simulink model "P4_Model_Final"  (R2023b)
settings: Solver=VariableStepAuto  StartTime=0.0  StopTime=3600  RelTol=1e-3
values from neighbouring files (symbols this model uses):
  C0 = 0.0041    [P4initUpdated.m]
  C1 = 0.000066    (= 6.6e-05)    [P4initUpdated.m]
  C2 = 0.5*Rho*A*Cd    (= 0.51156)    [P4initUpdated.m]
  Iw = 0.5*7*(r^2)    (= 0.4536)    [P4initUpdated.m]
  M = 1000    [P4initUpdated.m]
  r = 0.36    [P4initUpdated.m]
  rps2rpm = 60/(2*pi())    [P4initUpdated.m]
  Wp = [transpose(x), transpose(y)]    [genTrack.m]
undefined symbols (not defined in the file or in its folder): batData, carData, motorData
libraries: slpidlib x2
settings Model: Creator=jessi  LastModifiedBy=lmend

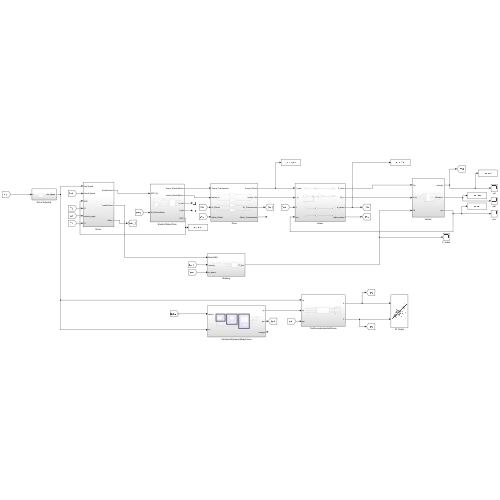
[thumbnail: Simulink's stored preview of the top-level diagram]
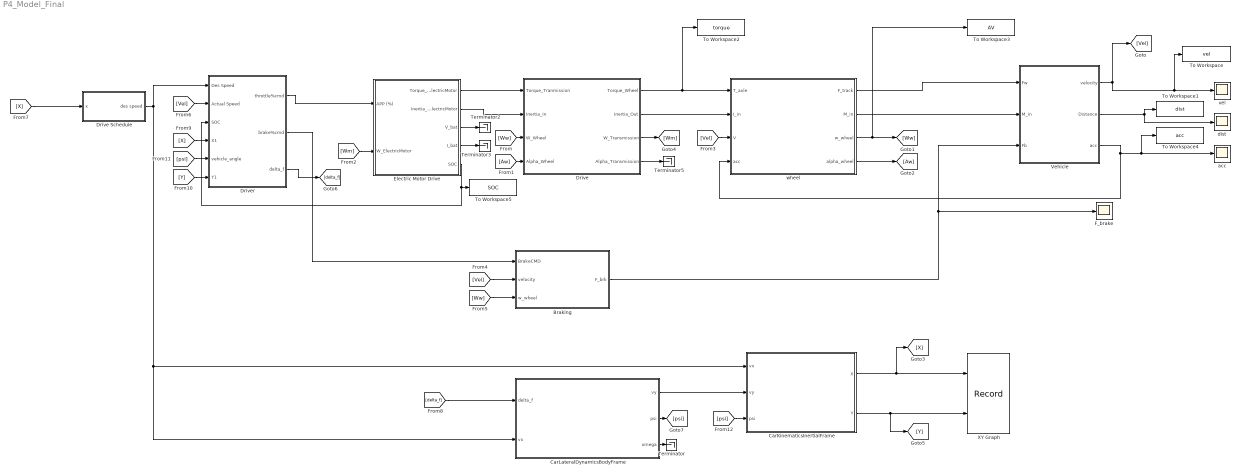
== system P4_Model_Final ==
  Braking : Subsystem
  CarKinematicsInertialFrame : Subsystem
  CarLateralDynamicsBodyFrame : Subsystem
  Drive : Subsystem
  Drive Schedule : Subsystem
  Driver : Subsystem
  Electric Motor Drive : Subsystem
  F_brake : Scope
  Terminator{,2..3,5} (4 alike) : Terminator
  To Workspace : ToWorkspace  VariableName=vel  SaveFormat=Timeseries  SampleTime=-1
  To Workspace1 : ToWorkspace  VariableName=dist  SaveFormat=Timeseries  SampleTime=-1
  To Workspace2 : ToWorkspace  VariableName=torque  SaveFormat=Timeseries  SampleTime=-1
  To Workspace3 : ToWorkspace  VariableName=AV  SaveFormat=Timeseries  SampleTime=-1
  To Workspace4 : ToWorkspace  VariableName=acc  SaveFormat=Timeseries  SampleTime=-1
  To Workspace5 : ToWorkspace  VariableName=SOC  SaveFormat=Timeseries  SampleTime=-1
  Vehicle : Subsystem
  XY Graph : Record  FileSettingsInternal="{\"entries\":[{\"content\":{\"excelSettings\":{\"content\":{},\"type\":\"Streamout.ExcelSettings\"}},\"type\":\"Streamout.FileSettingStorage\",\"uuid\":\"\"}],\"packageUris\":[\"http:\\/\\/schema.mathworks.com\\/mf0\\/streamout_blocks\\/R2020a\"],\"version\":\"1.0\"}"  Layout=[1 1]  SignalsInternal="{\"entries\":[{\"content\":{\"signals\":[{\"content\":{\"blockPath\":[],\"dimensions\":[1],\"domain\":\"\",\"lineColor\":\"#7e2f8e\",\"port\":1,\"sid\":[\"\"],\"signalID\":5613,\"signalName\":\"CarKinematicsInertialFrame:1\"},\"type\":\"RecordBlkView.Signal\",\"uuid\":\"\"},{\"content\":{\"blockPath\":[],\"dimensions\":[1],\"domain\":\"\",\"lineColor\":\"#77ac30\",\"port\":2,\"sid\":[\"\"],\"signalID\":5617,\"signalName\":\"CarKinematicsInertialFrame:2\"},\"type\":\"RecordBlkView.Signal\",\"uuid\":\"\"}]},\"type\":\"RecordBlkView.InputSignals\",\"uuid\":\"\"}],\"packageUris\":[\"http:\\/\\/schema.mathworks.com\\/mf0\\/streamout_blocks\\/R2020a\"],\"version\":\"1.0\"}"  VisualizationBindings="{\"xyplotplugin\":{\"info\":[{\"series\":[],\"subplotID\":1}]}}"  CompatibilityTag=XY  st=-1
  acc : Scope
  dist : Scope
  vel : Scope
  "wheel " : Subsystem
  wires:
  [Ww] -> Braking/3(w_wheel)
  [Vel] -> Braking/2("velocity ")
  "wheel "/3(w_wheel) -> To Workspace3/1, [Ww]
  "wheel "/1(F_track) -> Vehicle/1("Fw ")
  [Wm] -> Electric Motor Drive/2(W_ElectricMotor)
  "wheel "/2(M_in) -> Vehicle/2("M_in ")
  [Ww] -> Drive/3(W_Wheel)
  Drive/1(Torque_Wheel) -> To Workspace2/1, "wheel "/1(T_axle)
  Drive/2(Inertia_Out) -> "wheel "/2(I_in)
  Electric Motor Drive/4(I_bat) -> Terminator3/1
  [Vel] -> "wheel "/3(V)
  Electric Motor Drive/3(V_bat) -> Terminator2/1
  Vehicle/2("Distance ") -> dist/1, To Workspace1/1
  Braking/1("F_brk ") -> F_brake/1, Vehicle/3("Fb ")
  Drive/4(Alpha_Transmission) -> Terminator5/1
  Electric Motor Drive/2(Inertia_ElectricMotor) -> Drive/2(Inertia_In)
  Vehicle/3(acc) -> "wheel "/4(acc), To Workspace4/1, acc/1
  Vehicle/1("velocity ") -> To Workspace/1, vel/1, [Vel]
  Electric Motor Drive/1(Torque_ElectricMotor) -> Drive/1(Torque_Tranmission)
  "wheel "/4(alpha_wheel) -> [Aw]
  [Aw] -> Drive/4(Alpha_Wheel)
  Drive/3(W_Transmission) -> [Wm]
  Drive Schedule/1("des speed ") -> Driver/1("Des Speed "), CarKinematicsInertialFrame/1(vx), CarLateralDynamicsBodyFrame/2(vx)
  [delta_f] -> CarLateralDynamicsBodyFrame/1(delta_f)
  CarKinematicsInertialFrame/1(X) -> [X], XY Graph/1
  CarKinematicsInertialFrame/2(Y) -> [Y], XY Graph/2
  CarLateralDynamicsBodyFrame/1(vy) -> CarKinematicsInertialFrame/2(vy)
  [X] -> Drive Schedule/1(x)
  CarLateralDynamicsBodyFrame/3(omega) -> Terminator/1
  [Y] -> Driver/6(Y1)
  Driver/3(delta_f) -> [delta_f]
  Driver/2("brake%cmd ") -> Braking/1("BrakeCMD ")
  Driver/1(throttle%cmd) -> Electric Motor Drive/1(APP (%))
  CarLateralDynamicsBodyFrame/2(psi) -> [psi]
  [psi] -> CarKinematicsInertialFrame/3(psi)
  Electric Motor Drive/5(SOC) -> Driver/3(SOC), To Workspace5/1
  [X] -> Driver/4(X1)
  [Vel] -> Driver/2(Actual Speed)
  [psi] -> Driver/5(vehicle_angle)

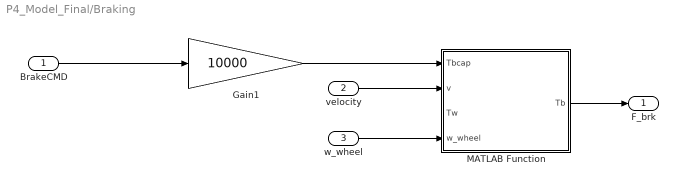
== system P4_Model_Final/Braking ==
  "BrakeCMD " : Inport
  "velocity " : Inport  Port=2
  w_wheel : Inport  Port=3
  Gain1 : Gain  Gain=10000
  MATLAB Function : MATLAB Function  TreatAsAtomicUnit=on
  "F_brk " : Outport  VectorParamsAs1DForOutWhenUnconnected=off
  wires:
  "BrakeCMD "/1 -> Gain1/1
  Gain1/1 -> MATLAB Function/1(Tbcap)
  MATLAB Function/1(Tb) -> "F_brk "/1
  "velocity "/1 -> MATLAB Function/2(v)
  w_wheel/1 -> MATLAB Function/4(w_wheel)

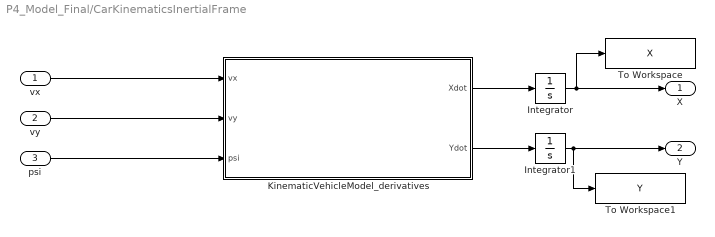
== system P4_Model_Final/CarKinematicsInertialFrame ==
  vx : Inport
  vy : Inport  Port=2
  psi : Inport  Port=3
  Integrator : Integrator  InitialCondition=carData.init.X0
  Integrator1 : Integrator  InitialCondition=carData.init.Y0
  KinematicVehicleModel_derivatives : MATLAB Function  TreatAsAtomicUnit=on  mask{obj=carData}
      mask prompts: obj "obj structure"
  To Workspace : ToWorkspace  VariableName=X  SaveFormat=Timeseries  SampleTime=-1
  To Workspace1 : ToWorkspace  VariableName=Y  SaveFormat=Timeseries  SampleTime=-1
  X : Outport
  Y : Outport  Port=2
  wires:
  KinematicVehicleModel_derivatives/1(Xdot) -> Integrator/1
  KinematicVehicleModel_derivatives/2(Ydot) -> Integrator1/1
  Integrator/1 -> To Workspace/1, X/1
  Integrator1/1 -> To Workspace1/1, Y/1
  vx/1 -> KinematicVehicleModel_derivatives/1(vx)
  vy/1 -> KinematicVehicleModel_derivatives/2(vy)
  psi/1 -> KinematicVehicleModel_derivatives/3(psi)

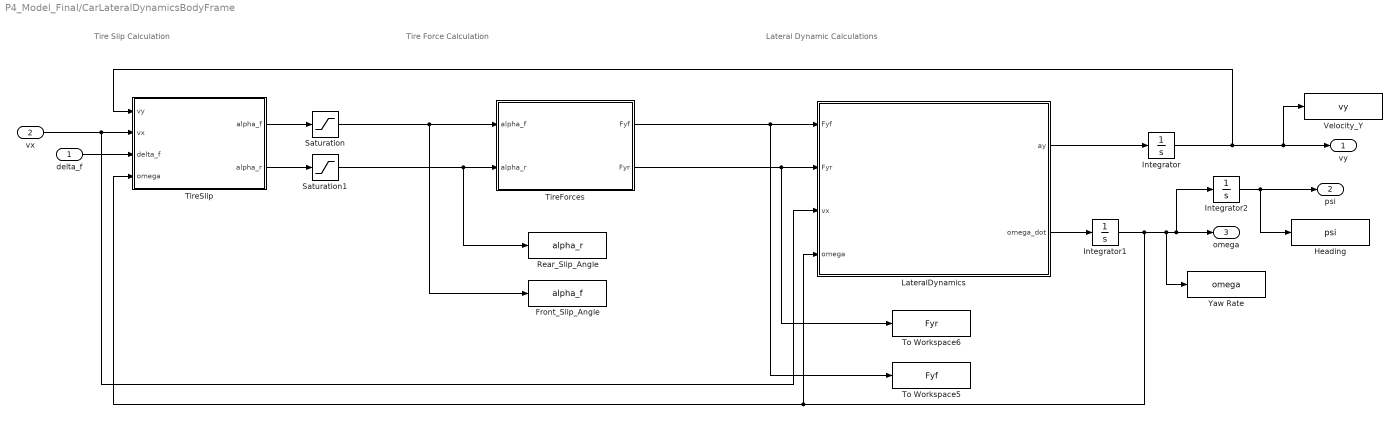
== system P4_Model_Final/CarLateralDynamicsBodyFrame ==
  note: Tire Slip Calculation
  note: Tire Force Calculation
  note: Lateral Dynamic Calculations
  delta_f : Inport
  vx : Inport  Port=2
  Front_Slip_Angle : ToWorkspace  VariableName=alpha_f  SaveFormat=Timeseries  SampleTime=-1
  Heading : ToWorkspace  VariableName=psi  SaveFormat=Timeseries  SampleTime=-1
  Integrator : Integrator  InitialCondition=carData.init.vy0
  Integrator1 : Integrator  InitialCondition=carData.init.omega0
  Integrator2 : Integrator  InitialCondition=carData.init.psi0
  LateralDynamics : MATLAB Function  TreatAsAtomicUnit=on  mask{obj=carData}
      mask prompts: obj "obj structure"
  Rear_Slip_Angle : ToWorkspace  VariableName=alpha_r  SaveFormat=Timeseries  SampleTime=-1
  Saturation : Saturate  UpperLimit=carData.maxAlpha  LowerLimit=-carData.maxAlpha
  Saturation1 : Saturate  UpperLimit=carData.maxAlpha  LowerLimit=-carData.maxAlpha
  TireForces : MATLAB Function  TreatAsAtomicUnit=on  mask{obj=carData}
      mask prompts: obj "obj structure"
  TireSlip : MATLAB Function  TreatAsAtomicUnit=on  mask{obj=carData}
      mask prompts: obj "obj structure"
  To Workspace5 : ToWorkspace  VariableName=Fyf  SaveFormat=Timeseries  SampleTime=-1
  To Workspace6 : ToWorkspace  VariableName=Fyr  SaveFormat=Timeseries  SampleTime=-1
  Velocity_Y : ToWorkspace  VariableName=vy  SaveFormat=Timeseries  SampleTime=-1
  Yaw Rate : ToWorkspace  VariableName=omega  SaveFormat=Timeseries  SampleTime=-1
  vy : Outport
  psi : Outport  Port=2
  omega : Outport  Port=3
  wires:
  LateralDynamics/1(ay) -> Integrator/1
  Integrator/1 -> vy/1, Velocity_Y/1, TireSlip/1(vy)
  LateralDynamics/2(omega_dot) -> Integrator1/1
  Integrator1/1 -> Integrator2/1, omega/1, Yaw Rate/1, LateralDynamics/4(omega), TireSlip/4(omega)
  TireSlip/1(alpha_f) -> Saturation/1
  TireSlip/2(alpha_r) -> Saturation1/1
  TireForces/1(Fyf) -> LateralDynamics/1(Fyf), To Workspace5/1
  TireForces/2(Fyr) -> LateralDynamics/2(Fyr), To Workspace6/1
  Saturation/1 -> TireForces/1(alpha_f), Front_Slip_Angle/1
  Saturation1/1 -> TireForces/2(alpha_r), Rear_Slip_Angle/1
  vx/1 -> TireSlip/2(vx), LateralDynamics/3(vx)
  delta_f/1 -> TireSlip/3(delta_f)
  Integrator2/1 -> Heading/1, psi/1

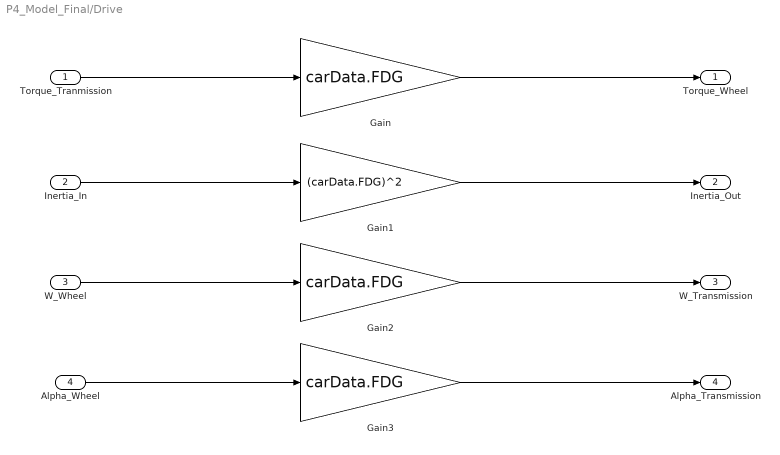
== system P4_Model_Final/Drive ==
  Torque_Tranmission : Inport
  Inertia_In : Inport  Port=2
  W_Wheel : Inport  Port=3
  Alpha_Wheel : Inport  Port=4
  Gain : Gain  Gain=carData.FDG
  Gain1 : Gain  Gain=(carData.FDG)^2
  Gain2 : Gain  Gain=carData.FDG
  Gain3 : Gain  Gain=carData.FDG
  Torque_Wheel : Outport
  Inertia_Out : Outport  Port=2
  W_Transmission : Outport  Port=3
  Alpha_Transmission : Outport  Port=4
  wires:
  Torque_Tranmission/1 -> Gain/1
  Inertia_In/1 -> Gain1/1
  W_Wheel/1 -> Gain2/1
  Alpha_Wheel/1 -> Gain3/1
  Gain/1 -> Torque_Wheel/1
  Gain1/1 -> Inertia_Out/1
  Gain2/1 -> W_Transmission/1
  Gain3/1 -> Alpha_Transmission/1

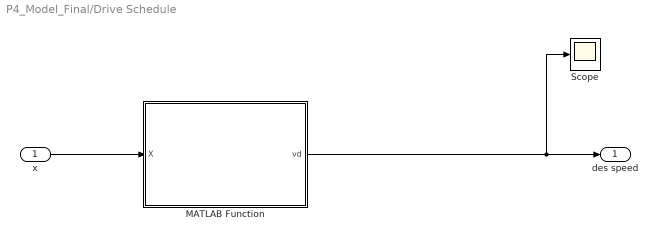
== system P4_Model_Final/Drive Schedule ==
  x : Inport
  MATLAB Function : MATLAB Function  TreatAsAtomicUnit=on
  Scope : Scope
  "des speed " : Outport  VectorParamsAs1DForOutWhenUnconnected=off
  wires:
  x/1 -> MATLAB Function/1(X)
  MATLAB Function/1(vd) -> "des speed "/1, Scope/1

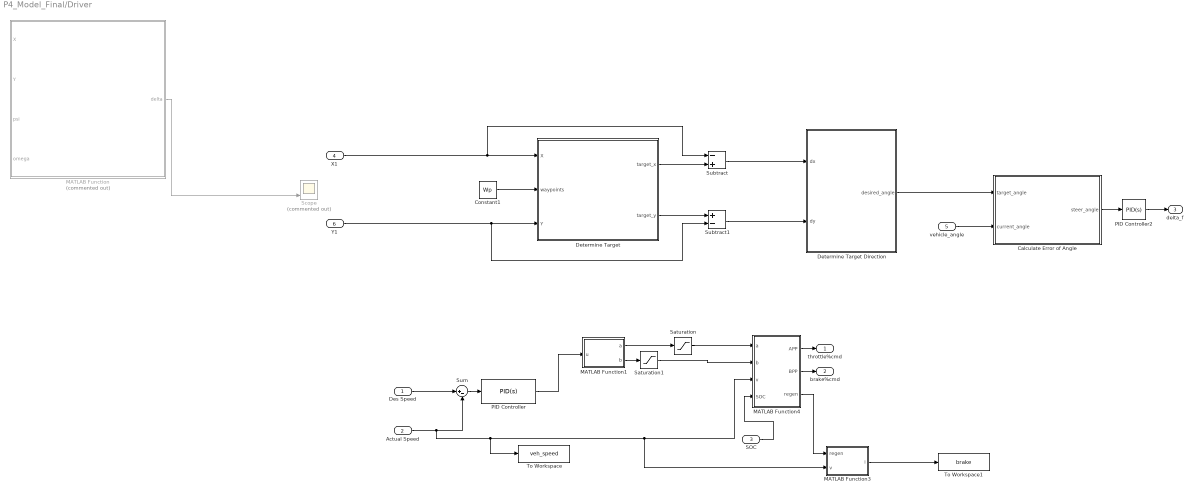
== system P4_Model_Final/Driver ==
  "Des Speed " : Inport
  Actual Speed : Inport  Port=2
  SOC : Inport  Port=3
  X1 : Inport  Port=4
  vehicle_angle : Inport  Port=5
  Y1 : Inport  Port=6
  Calculate Error of Angle : MATLAB Function  TreatAsAtomicUnit=on
  Constant1 : Constant  Value=Wp
  Determine Target : MATLAB Function  TreatAsAtomicUnit=on
  Determine Target Direction : MATLAB Function  TreatAsAtomicUnit=on
  MATLAB Function : MATLAB Function  Commented=on  TreatAsAtomicUnit=on
  MATLAB Function1 : MATLAB Function  TreatAsAtomicUnit=on
  MATLAB Function3 : MATLAB Function  TreatAsAtomicUnit=on
  MATLAB Function4 : MATLAB Function  TreatAsAtomicUnit=on
  PID Controller : slpidlib/PID Controller  Controller=PID  Form=Parallel  TimeDomain=Continuous-time  UseExternalTs=off  SampleTime=-1  IntegratorMethod=Forward Euler  FilterMethod=Forward Euler  ControllerParametersSource=internal  P=0.55  I=0  UseKiTs=off  D=0  N=100  UseFilter=on  TunerSelectOption=Transfer Function Based (PID Tuner App)  InitialConditionSource=internal  InitialConditionForIntegrator=0  InitialConditionForFilter=0  DifferentiatorICPrevScaledInput=0  ExternalReset=none  TrackingMode=off  Kt=1  LimitOutput=on  SatLimitsSource=internal  UpperSaturationLimit=1  LowerSaturationLimit=-1  LinearizeAsGain=off  AntiWindupMode=none  Kb=1  LimitIntegrator=off  UpperIntegratorSaturationLimit=inf  LowerIntegratorSaturationLimit=-inf  POutMin=[]  POutMax=[]  IOutMin=[]  IOutMax=[]  DOutMin=[]  DOutMax=[]  NOutMin=[]  NOutMax=[]  SumOutMin=[]  SumOutMax=[]  SaturationOutMin=[]  SaturationOutMax=[]  PParamMin=[]  PParamMax=[]  IParamMin=[]  IParamMax=[]  DParamMin=[]  DParamMax=[]  NParamMin=[]  NParamMax=[]  KbParamMin=[]  KbParamMax=[]  KtParamMin=[]  KtParamMax=[]  KbOutMin=[]  KbOutMax=[]  KtOutMin=[]  KtOutMax=[]  IntegratorOutMin=[]  IntegratorOutMax=[]  FilterOutMin=[]  FilterOutMax=[]  SumI1OutMin=[]  SumI1OutMax=[]  SumI2OutMin=[]  SumI2OutMax=[]  SumI3OutMin=[]  SumI3OutMax=[]  SumI4OutMin=[]  SumI4OutMax=[]  SumDOutMin=[]  SumDOutMax=[]  DifferentiatorOutMin=[]  DifferentiatorOutMax=[]  FilterDiffOutCoefMin=[]  FilterDiffOutCoefMax=[]  ReciprocalOutMin=[]  ReciprocalOutMax=[]  SumDenOutMin=[]  SumDenOutMax=[]  SumNumOutMin=[]  SumNumOutMax=[]  DivideOutMin=[]  DivideOutMax=[]  UdiffTsProdOutMin=[]  UdiffTsProdOutMax=[]  NTsProdOutMin=[]  NTsProdOutMax=[]  UintegralTsProdOutMin=[]  UintegralTsProdOutMax=[]  UngainTsProdOutMin=[]  UngainTsProdOutMax=[]  ClampingZeroOutDataTypeStr=Inherit: Inherit via back propagation  ClampingZeroOutMin=[]  ClampingZeroOutMax=[]  FilterDenConstantOutDataTypeStr=Inherit: Inherit via back propagation  FilterDenConstantOutMin=[]  FilterDenConstantOutMax=[]  PCopyOutDataTypeStr=Inherit: Inherit via back propagation  PCopyOutMin=[]  PCopyOutMax=[]  NCopyOutDataTypeStr=Inherit: Inherit via back propagation  NCopyOutMin=[]  NCopyOutMax=[]  IntegratorContinuousStateAttributes=''  IntegratorStateMustResolveToSignalObject=off  IntegratorRTWStateStorageClass=Auto  FilterContinuousStateAttributes=''  FilterStateMustResolveToSignalObject=off  FilterRTWStateStorageClass=Auto  ParallelPVariant=InternalParameters  IdealPVariant=Disabled  IVariant=InternalParameters  DVariant=InternalParameters  IntegratorVariant=Continuous  SatVariant=Enabled  AWVariant=Passthrough  PCopyVariant=Disabled  TRVariant=Disabled  FdbkBlocksVariant=Forward  IdealPFdbkVariant=Disabled  SatFdbkVariant=Disabled  DerivativeFilterVariant=ContFilter  NVariant=InternalParameters  NCopyVariant=Disabled  FilterICVariant=InternalICsFilter  IntegratorICVariant=InternalICs  ExternalResetVariant=Disabled  TRSumVariant=Passthrough  SumFdbkVariant=Disabled  SumVariant=Sum_PID  TsampFilterVariant=InternalTs  TsampNgainVariant=Passthrough  TsampIntegralVariant=Disabled_SignalSpec  ExternalSaturationOutDataTypeStr=Inherit: Same as second input
  PID Controller2 : slpidlib/PID Controller  Controller=PID  Form=Parallel  TimeDomain=Continuous-time  UseExternalTs=off  SampleTime=-1  IntegratorMethod=Forward Euler  FilterMethod=Forward Euler  ControllerParametersSource=internal  P=1  I=0.1  UseKiTs=off  D=0  N=100  UseFilter=on  TunerSelectOption=Transfer Function Based (PID Tuner App)  InitialConditionSource=internal  InitialConditionForIntegrator=0  InitialConditionForFilter=0  DifferentiatorICPrevScaledInput=0  ExternalReset=none  TrackingMode=off  Kt=1  LimitOutput=off  SatLimitsSource=internal  UpperSaturationLimit=inf  LowerSaturationLimit=-inf  LinearizeAsGain=on  AntiWindupMode=none  Kb=1  LimitIntegrator=off  UpperIntegratorSaturationLimit=inf  LowerIntegratorSaturationLimit=-inf  POutMin=[]  POutMax=[]  IOutMin=[]  IOutMax=[]  DOutMin=[]  DOutMax=[]  NOutMin=[]  NOutMax=[]  SumOutMin=[]  SumOutMax=[]  SaturationOutMin=[]  SaturationOutMax=[]  PParamMin=[]  PParamMax=[]  IParamMin=[]  IParamMax=[]  DParamMin=[]  DParamMax=[]  NParamMin=[]  NParamMax=[]  KbParamMin=[]  KbParamMax=[]  KtParamMin=[]  KtParamMax=[]  KbOutMin=[]  KbOutMax=[]  KtOutMin=[]  KtOutMax=[]  IntegratorOutMin=[]  IntegratorOutMax=[]  FilterOutMin=[]  FilterOutMax=[]  SumI1OutMin=[]  SumI1OutMax=[]  SumI2OutMin=[]  SumI2OutMax=[]  SumI3OutMin=[]  SumI3OutMax=[]  SumI4OutMin=[]  SumI4OutMax=[]  SumDOutMin=[]  SumDOutMax=[]  DifferentiatorOutMin=[]  DifferentiatorOutMax=[]  FilterDiffOutCoefMin=[]  FilterDiffOutCoefMax=[]  ReciprocalOutMin=[]  ReciprocalOutMax=[]  SumDenOutMin=[]  SumDenOutMax=[]  SumNumOutMin=[]  SumNumOutMax=[]  DivideOutMin=[]  DivideOutMax=[]  UdiffTsProdOutMin=[]  UdiffTsProdOutMax=[]  NTsProdOutMin=[]  NTsProdOutMax=[]  UintegralTsProdOutMin=[]  UintegralTsProdOutMax=[]  UngainTsProdOutMin=[]  UngainTsProdOutMax=[]  ClampingZeroOutDataTypeStr=Inherit: Inherit via back propagation  ClampingZeroOutMin=[]  ClampingZeroOutMax=[]  FilterDenConstantOutDataTypeStr=Inherit: Inherit via back propagation  FilterDenConstantOutMin=[]  FilterDenConstantOutMax=[]  PCopyOutDataTypeStr=Inherit: Inherit via back propagation  PCopyOutMin=[]  PCopyOutMax=[]  NCopyOutDataTypeStr=Inherit: Inherit via back propagation  NCopyOutMin=[]  NCopyOutMax=[]  IntegratorContinuousStateAttributes=''  IntegratorStateMustResolveToSignalObject=off  IntegratorRTWStateStorageClass=Auto  FilterContinuousStateAttributes=''  FilterStateMustResolveToSignalObject=off  FilterRTWStateStorageClass=Auto  ParallelPVariant=InternalParameters  IdealPVariant=Disabled  IVariant=InternalParameters  DVariant=InternalParameters  IntegratorVariant=Continuous  SatVariant=Disabled  AWVariant=Passthrough  PCopyVariant=Disabled  TRVariant=Disabled  FdbkBlocksVariant=Forward  IdealPFdbkVariant=Disabled  SatFdbkVariant=Disabled  DerivativeFilterVariant=ContFilter  NVariant=InternalParameters  NCopyVariant=Disabled  FilterICVariant=InternalICsFilter  IntegratorICVariant=InternalICs  ExternalResetVariant=Disabled  TRSumVariant=Passthrough  SumFdbkVariant=Disabled  SumVariant=Sum_PID  TsampFilterVariant=InternalTs  TsampNgainVariant=Passthrough  TsampIntegralVariant=Disabled_SignalSpec  ExternalSaturationOutDataTypeStr=Inherit: Same as second input
  Saturation : Saturate  UpperLimit=1  LowerLimit=0
  Saturation1 : Saturate  UpperLimit=0  LowerLimit=-1
  Scope : Scope  Commented=on  NumInputPorts=3
  Subtract : Sum  Inputs=-+
  Subtract1 : Sum  Inputs=+-
  Sum : Sum  Inputs=|+-
  To Workspace : ToWorkspace  VariableName=veh_speed  SaveFormat=Timeseries  SampleTime=-1
  To Workspace1 : ToWorkspace  VariableName=brake  SaveFormat=Timeseries  SampleTime=-1
  throttle%cmd : Outport
  "brake%cmd " : Outport  Port=2
  delta_f : Outport  Port=3
  wires:
  MATLAB Function/1(delta) -> Scope/3
  PID Controller/1 -> MATLAB Function1/1(u)
  MATLAB Function1/2(b) -> Saturation1/1
  Actual Speed/1 -> To Workspace/1, MATLAB Function3/2(v), MATLAB Function4/3(v), Sum/2
  Sum/1 -> PID Controller/1
  MATLAB Function1/1(a) -> Saturation/1
  "Des Speed "/1 -> Sum/1
  MATLAB Function3/1(i) -> To Workspace1/1
  MATLAB Function4/2(BPP) -> "brake%cmd "/1
  MATLAB Function4/1(APP) -> throttle%cmd/1
  MATLAB Function4/3(regen) -> MATLAB Function3/1(regen)
  Saturation/1 -> MATLAB Function4/1(a)
  Saturation1/1 -> MATLAB Function4/2(b)
  SOC/1 -> MATLAB Function4/4(SOC)
  Determine Target/1(target_x) -> Subtract/2
  Y1/1 -> Subtract1/2, Determine Target/3(Y)
  Subtract1/1 -> Determine Target Direction/2(dy)
  Determine Target Direction/1(desired_angle) -> Calculate Error of Angle/1(target_angle)
  Determine Target/2(target_y) -> Subtract1/1
  Constant1/1 -> Determine Target/2(waypoints)
  Subtract/1 -> Determine Target Direction/1(dx)
  PID Controller2/1 -> delta_f/1
  X1/1 -> Subtract/1, Determine Target/1(X)
  vehicle_angle/1 -> Calculate Error of Angle/2(current_angle)
  Calculate Error of Angle/1(steer_angle) -> PID Controller2/1

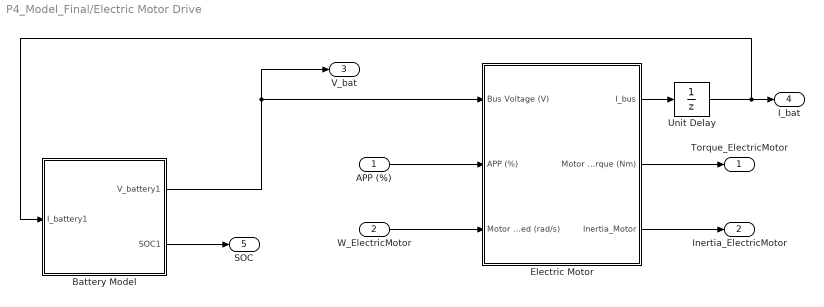
== system P4_Model_Final/Electric Motor Drive ==
  APP (%) : Inport
  W_ElectricMotor : Inport  Port=2
  Battery Model : Subsystem  TreatAsAtomicUnit=on
  Electric Motor : Subsystem  TreatAsAtomicUnit=on
  Unit Delay : UnitDelay  SampleTime=-1  HasFrameUpgradeWarning=on
  Torque_ElectricMotor : Outport
  Inertia_ElectricMotor : Outport  Port=2
  V_bat : Outport  Port=3
  I_bat : Outport  Port=4
  SOC : Outport  Port=5
  wires:
  Electric Motor/2(Motor Torque (Nm)) -> Torque_ElectricMotor/1
  Battery Model/2(SOC1) -> SOC/1
  Electric Motor/3(Inertia_Motor) -> Inertia_ElectricMotor/1
  W_ElectricMotor/1 -> Electric Motor/3(Motor Speed (rad/s))
  Electric Motor/1(I_bus) -> Unit Delay/1
  APP (%)/1 -> Electric Motor/2(APP (%))
  Battery Model/1(V_battery1) -> Electric Motor/1(Bus Voltage (V)), V_bat/1
  Unit Delay/1 -> Battery Model/1(I_battery1), I_bat/1

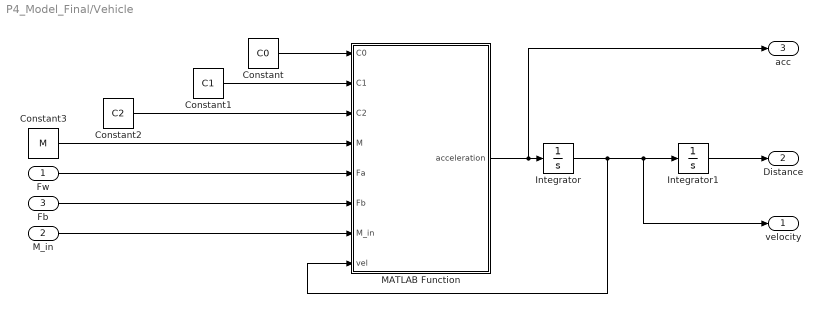
== system P4_Model_Final/Vehicle ==
  "Fw " : Inport
  "M_in " : Inport  Port=2
  "Fb " : Inport  Port=3
  Constant : Constant  Value=C0
  Constant1 : Constant  Value=C1
  Constant2 : Constant  Value=C2
  Constant3 : Constant  Value=M
  Integrator : Integrator  LimitOutput=on  LowerSaturationLimit=0
  Integrator1 : Integrator
  MATLAB Function : MATLAB Function  TreatAsAtomicUnit=on
  "velocity " : Outport  VectorParamsAs1DForOutWhenUnconnected=off
  "Distance " : Outport  Port=2  VectorParamsAs1DForOutWhenUnconnected=off
  acc : Outport  Port=3
  wires:
  Constant1/1 -> MATLAB Function/2(C1)
  Constant/1 -> MATLAB Function/1(C0)
  MATLAB Function/1(acceleration) -> acc/1, Integrator/1
  Constant2/1 -> MATLAB Function/3(C2)
  Constant3/1 -> MATLAB Function/4(M)
  "Fw "/1 -> MATLAB Function/5(Fa)
  "Fb "/1 -> MATLAB Function/6(Fb)
  Integrator/1 -> MATLAB Function/8(vel), "velocity "/1, Integrator1/1
  Integrator1/1 -> "Distance "/1
  "M_in "/1 -> MATLAB Function/7(M_in)

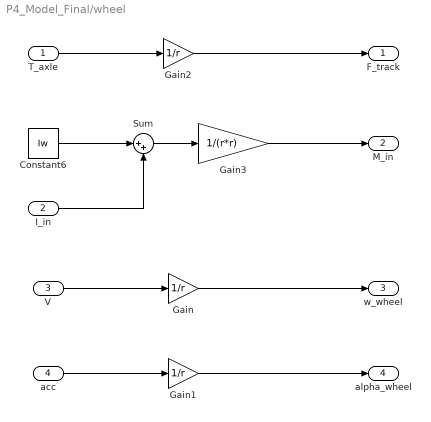
== system P4_Model_Final/wheel  ==
  T_axle : Inport
  I_in : Inport  Port=2
  V : Inport  Port=3
  acc : Inport  Port=4
  Constant6 : Constant  Value=Iw
  Gain : Gain  Gain=1/r
  Gain1 : Gain  Gain=1/r
  Gain2 : Gain  Gain=1/r
  Gain3 : Gain  Gain=1/(r*r)
  Sum : Sum  Inputs=|++
  F_track : Outport
  M_in : Outport  Port=2
  w_wheel : Outport  Port=3
  alpha_wheel : Outport  Port=4
  wires:
  Gain/1 -> w_wheel/1
  V/1 -> Gain/1
  acc/1 -> Gain1/1
  Gain1/1 -> alpha_wheel/1
  T_axle/1 -> Gain2/1
  Gain2/1 -> F_track/1
  Gain3/1 -> M_in/1
  Constant6/1 -> Sum/1
  I_in/1 -> Sum/2
  Sum/1 -> Gain3/1

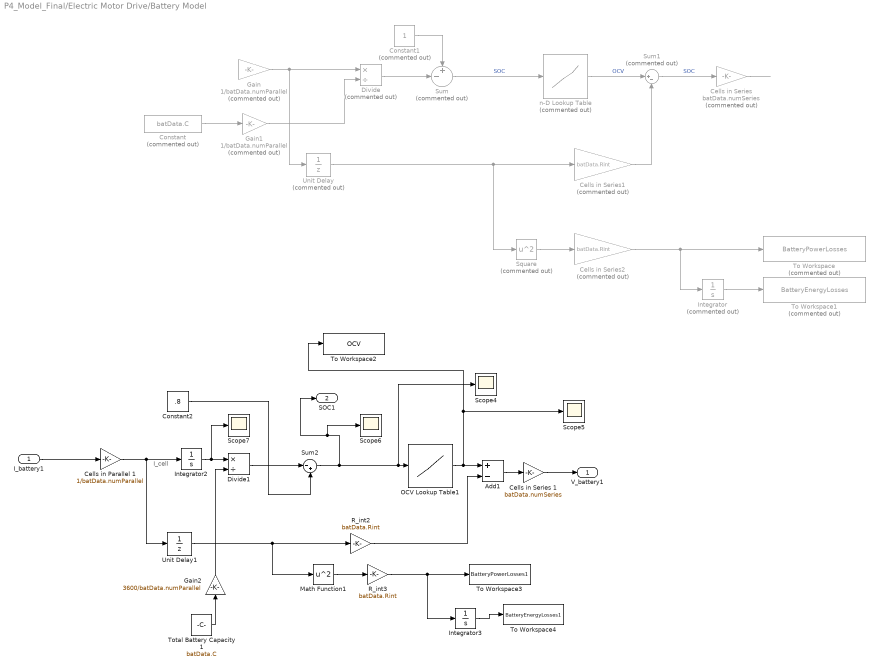
== system P4_Model_Final/Electric Motor Drive/Battery Model ==
  note: I_cell
  I_battery1 : Inport
  Add1 : Sum  Inputs=+-
  Cells in Parallel 1 : Gain  Gain=1/batData.numParallel
  Cells in Series : Gain  Commented=on  Gain=batData.numSeries
  Cells in Series 1 : Gain  Gain=batData.numSeries
  Cells in Series1 : Gain  Commented=on  Gain=batData.Rint
  Cells in Series2 : Gain  Commented=on  Gain=batData.Rint
  Constant : Constant  Commented=on  Value=batData.C
  Constant1 : Constant  Commented=on
  Constant2 : Constant  Value=.8
  Divide : Product  Commented=on  Inputs=*/
  Divide1 : Product  Inputs=*/
  Gain : Gain  Commented=on  Gain=1/batData.numParallel
  Gain1 : Gain  Commented=on  Gain=1/batData.numParallel
  Gain2 : Gain  Gain=3600/batData.numParallel
  Integrator : Integrator  Commented=on
  Integrator2 : Integrator
  Integrator3 : Integrator
  Math Function1 : Math  Operator=square
  OCV Lookup Table1 : Lookup_n-D  NumberOfTableDimensions=1  LookupTableObject=''  BreakpointsForDimension1=batData.SOC  BreakpointsForDimension2FirstPoint=10  BreakpointsForDimension1Spacing=12  BreakpointsForDimension2Spacing=12  Table=batData.OCV  InterpMethod=Flat  ExtrapMethod=Cubic spline  RemoveProtectionInput=on  InternalRulePriority=Speed  RndMeth=Simplest
  R_int2 : Gain  Gain=batData.Rint
  R_int3 : Gain  Gain=batData.Rint
  Scope{4..7} (4 alike) : Scope
  Square : Math  Commented=on  Operator=square
  Sum : Sum  Commented=on  Inputs=+-|
  Sum1 : Sum  Commented=on  Inputs=|+-
  Sum2 : Sum  Inputs=|-+
  To Workspace : ToWorkspace  Commented=on  VariableName=BatteryPowerLosses  SaveFormat=Timeseries  SampleTime=-1
  To Workspace1 : ToWorkspace  Commented=on  VariableName=BatteryEnergyLosses  SaveFormat=Timeseries  SampleTime=-1
  To Workspace2 : ToWorkspace  VariableName=OCV  SaveFormat=Timeseries  SampleTime=-1
  To Workspace3 : ToWorkspace  VariableName=BatteryPowerLosses1  SaveFormat=Timeseries  SampleTime=-1
  To Workspace4 : ToWorkspace  VariableName=BatteryEnergyLosses1  SaveFormat=Timeseries  SampleTime=-1
  Total Battery Capacity 1 : Constant  Value=batData.C
  Unit Delay : UnitDelay  Commented=on  SampleTime=-1  HasFrameUpgradeWarning=on
  Unit Delay1 : UnitDelay  SampleTime=-1  HasFrameUpgradeWarning=on
  n-D Lookup Table : Lookup_n-D  Commented=on  NumberOfTableDimensions=1  BreakpointsForDimension1=batData.SOC  BreakpointsForDimension3=[5, 7]  Table=batData.OCV  InternalRulePriority=Speed  RndMeth=Simplest
  V_battery1 : Outport
  SOC1 : Outport  Port=2
  wires:
  Gain/1 -> Unit Delay/1, Divide/1
  Gain1/1 -> Divide/2
  Constant/1 -> Gain1/1
  Constant1/1 -> Sum/1
  Divide/1 -> Sum/2
  Sum/1 -> n-D Lookup Table/1  "SOC"
  n-D Lookup Table/1 -> Sum1/1  "OCV"
  Cells in Series/1 -> ?
  Sum1/1 -> Cells in Series/1  "SOC"
  Cells in Series1/1 -> Sum1/2
  Square/1 -> Cells in Series2/1
  Cells in Series2/1 -> Integrator/1, To Workspace/1
  Integrator/1 -> To Workspace1/1
  Unit Delay/1 -> Square/1, Cells in Series1/1
  Add1/1 -> Cells in Series 1/1
  OCV Lookup Table1/1 -> To Workspace2/1, Scope5/1, Add1/1
  Unit Delay1/1 -> Math Function1/1, R_int2/1
  Math Function1/1 -> R_int3/1
  R_int2/1 -> Add1/2
  Divide1/1 -> Sum2/1
  I_battery1/1 -> Cells in Parallel 1/1
  R_int3/1 -> Integrator3/1, To Workspace3/1
  Integrator3/1 -> To Workspace4/1
  Constant2/1 -> Sum2/2
  Gain2/1 -> Divide1/2
  Integrator2/1 -> Scope7/1, Divide1/1
  Sum2/1 -> Scope4/1, OCV Lookup Table1/1, Scope6/1, SOC1/1
  Cells in Parallel 1/1 -> Unit Delay1/1, Integrator2/1
  Cells in Series 1/1 -> V_battery1/1
  Total Battery Capacity 1/1 -> Gain2/1

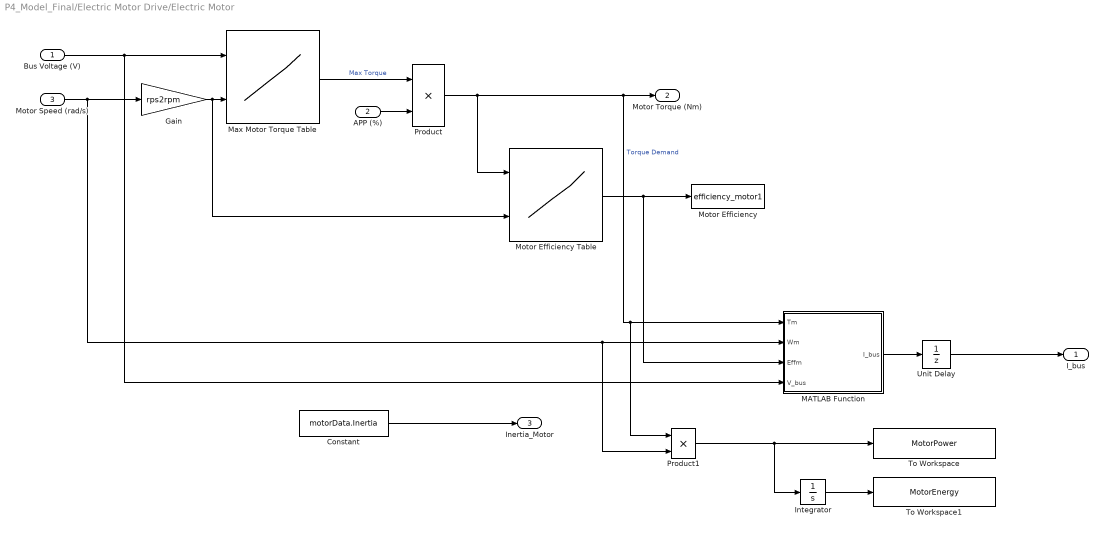
== system P4_Model_Final/Electric Motor Drive/Electric Motor ==
  Bus Voltage (V) : Inport
  APP (%) : Inport  Port=2
  Motor Speed (rad/s) : Inport  Port=3
  Constant : Constant  Value=motorData.Inertia
  Gain : Gain  Gain=rps2rpm
  Integrator : Integrator
  MATLAB Function : MATLAB Function  TreatAsAtomicUnit=on
  Max Motor Torque Table : Lookup_n-D  BreakpointsForDimension1=motorData.vbus  BreakpointsForDimension2=motorData.rpm  BreakpointsForDimension3=[5, 7]  Table=motorData.maxtorque  InternalRulePriority=Speed  RndMeth=Simplest
      settings: InputPortMap=u0,u1
  Motor Efficiency : ToWorkspace  VariableName=efficiency_motor1  SaveFormat=Timeseries  SampleTime=-1
  Motor Efficiency Table : Lookup_n-D  BreakpointsForDimension1=motorData.eta_torque  BreakpointsForDimension2=motorData.eta_speed  BreakpointsForDimension3=[5, 7]  Table=motorData.eta_val  InternalRulePriority=Speed  RndMeth=Simplest
      settings: InputPortMap=u0,u1
  Product : Product
  Product1 : Product
  To Workspace : ToWorkspace  VariableName=MotorPower  SaveFormat=Timeseries  SampleTime=-1
  To Workspace1 : ToWorkspace  VariableName=MotorEnergy  SaveFormat=Timeseries  SampleTime=-1
  Unit Delay : UnitDelay  SampleTime=-1  HasFrameUpgradeWarning=on
  I_bus : Outport
  Motor Torque (Nm) : Outport  Port=2
  Inertia_Motor : Outport  Port=3
  wires:
  Constant/1 -> Inertia_Motor/1
  APP (%)/1 -> Product/2
  Max Motor Torque Table/1 -> Product/1  "Max Torque"
  Product/1 -> Motor Efficiency Table/1, Product1/1, MATLAB Function/1(Tm), Motor Torque (Nm)/1  "Torque Demand"
  Gain/1 -> Motor Efficiency Table/2, Max Motor Torque Table/2
  Motor Speed (rad/s)/1 -> Gain/1, Product1/2, MATLAB Function/2(Wm)
  Motor Efficiency Table/1 -> MATLAB Function/3(Effm), Motor Efficiency/1
  Integrator/1 -> To Workspace1/1
  Product1/1 -> Integrator/1, To Workspace/1
  MATLAB Function/1(I_bus) -> Unit Delay/1
  Unit Delay/1 -> I_bus/1
  Bus Voltage (V)/1 -> MATLAB Function/4(V_bus), Max Motor Torque Table/1

== matlab function P4_Model_Final/Driver/MATLAB Function ==
  data: X input; delta output; Y input; psi input; omega input
function delta = SimplestDriver(X,Y,psi,omega)

if X > 900
    R = 200;
    L = pi*R;
    delta = L/R;
    
     
elseif X < 0
    R = 200;
    L = pi*R;
    delta = L/R;
    
elseif X < 900 && Y < 1
    delta = 0;


elseif X < 900 && X > 850 && Y > 390
    k = -0.00040;
    psi_d = 0;

    delta = k*(psi-psi_d);

else
    k = -0.00012;
    psi_d = 3;

    delta = k*(psi-psi_d);
end

== matlab function P4_Model_Final/Driver/MATLAB Function1 ==
  data: u input; a output; b output
% Checks if there is a difference between actual speed and desired speed

% u is calculated using the sum function in the simulink model

function [a,b] = fcn(u)

if u>0 % If the difference is greater than zero, then we need to speed up since actual speed is less than desired speed
    acc=u; % We send how much we need to speed up to the throttle command
    brk=0; % Do nothing for the break command
elseif u<0 % If the difference is less than zero, then we need to slow down since the actual speed is less than the desired speed
    acc=0; % Do nothing for throttle command
    brk=-u; % We send how much we need to break to the break command
else % If the desired and actual speed is the same
    acc=0; % Do nothing for throttle command
    brk=0; % Do nothing for the break command
end
a= acc; % storing how much acceleration required to a
b= brk; % storing how much break acceleration required to b

== matlab function P4_Model_Final/Driver/Calculate Error of Angle ==
  data: target_angle input; steer_angle output; current_angle input
function steer_angle = diff(target_angle, current_angle)

steer_angle = angdiff(current_angle, target_angle);

== matlab function P4_Model_Final/Driver/MATLAB Function3 ==
  data: regen input; i output; v input
function i = fcn(regen, v)
    speed = v * (3600 / 1600);
    if speed < 5
        regen_i = 0;
        if abs(regen - regen_i) < 1e-6
            i = 0;
        else
            i = 1;
        end
    
    elseif speed == 25
        regen_i = 0.95;
        if abs(regen - regen_i) < 1e-6
            i = 0;
        else
            i = 1;
        end
    
    elseif speed > 25
        regen_i = 0.95;
        if abs(regen - regen_i) < 1e-6
            i = 0;
        else
            i = 1;
        end
    else
        regen_i = (0.95/20)*speed - 0.2375;
        if abs(regen - regen_i) < 1e-6
            i = 0;
        else
            i = 1;
        end 
    end

== matlab function P4_Model_Final/Driver/MATLAB Function4 ==
  data: a input; APP output; BPP output; b input; v input; SOC input; regen output
function [APP, BPP, regen] = fcn(a, b, v, SOC)
    % Convert velocity to mph from m/s
    speed = v * (3600 / 1600);

    % Calculate regen based on speed and braking command
    regen = calculateRegen(speed);

    APP = a + b * regen;  % Add regen to the acceleration command
    BPP = b * (1 - regen);  % Rest is friction braking
end

function regen = calculateRegen(speed)
  if speed < 5
      regen = 0;
  elseif speed == 25
        regen = 0.95;
  elseif speed > 25
      regen = 0.95;
  else
      regen = ((0.95/20)*speed) - 0.2375;
  end 
end

== matlab function P4_Model_Final/Driver/Determine Target ==
  data: X input; waypoints input; Y input; target_x output; target_y output
function [target_x, target_y] = Driver(X, waypoints, Y)

waypoints = waypoints(1:end-1,:);

% Determine which waypoint is the closest
dist_from_waypoints_sqr = (waypoints(:,1)-X).^2+(waypoints(:,2)-Y).^2;
dist_from_waypoints = sqrt(dist_from_waypoints_sqr);

[~, idx] = min(dist_from_waypoints);

% Look ahead a few waypoints
target_idx = idx + 1;
if target_idx >= height(waypoints)
   target_idx = 1;
end
target_x = waypoints(target_idx,1);
target_y = waypoints(target_idx,2);

== matlab function P4_Model_Final/Drive Schedule/MATLAB Function ==
  data: X input; vd output
function vd = fcn(X)

if X > 0 && X < 900
    vd = 65;
else
    vd = 15;
end

== matlab function P4_Model_Final/Driver/Determine Target Direction ==
  data: dx input; desired_angle output; dy input
function desired_angle = fcn(dx,dy)

desired_angle = atan2(dy,dx);

% Make desired_angle a positive value always
if desired_angle < 0
    desired_angle = desired_angle + 2 * pi;
end

== matlab function P4_Model_Final/Vehicle/MATLAB Function ==
  data: C0 input; acceleration output; C1 input; C2 input; M input; Fa input; Fb input; M_in input; vel input
function acceleration   = vehicle(C0,C1,C2,M,Fa,Fb,M_in, vel)

acceleration = (((Fa-Fb))-(C0+ C1*vel + C2*(vel)^2))/(M+M_in);


% Fa: Force from wheel.
% Fb: Force from brake.
% -(C0+ C1*vel + C2*(vel)^2)): Force from drag (opposite direction of motion)

== matlab function P4_Model_Final/CarKinematicsInertialFrame/KinematicVehicleModel_derivatives ==
  data: vx input; vy input; psi input size=1; Xdot output; Ydot output
    function [Xdot, Ydot] = fcn(vx, vy, psi)
    temp = TF(psi) * [vx;vy]; 
    Xdot = temp(1);
    Ydot = temp(2);
  
end

function y = TF(psi)
    y = [cos(psi), -sin(psi); sin(psi), cos(psi)];
end

== matlab function P4_Model_Final/Electric Motor Drive/Electric Motor/MATLAB Function ==
  data: Tm input; I_bus output; Wm input; Effm input; V_bus input
function I_bus = fcn(Tm,Wm,Effm,V_bus)

%I_bus = (Tm*Wm/Effm)/V_bus;

Pm=Tm*Wm;
    if Pm >= 0
        sgn_m = 1;
    else
        sgn_m = -1;
    end
I_bus = ( (Pm) * (Effm)^(sgn_m) ) / V_bus;

== matlab function P4_Model_Final/CarLateralDynamicsBodyFrame/LateralDynamics ==
  data: Fyf input; Fyr input size=1; vx input; omega input; ay output; obj parameter; omega_dot output
function [ay, omega_dot] = fcn(Fyf, Fyr, vx, omega, obj)

Fy = Fyf + Fyr;
ay = Fy / obj.Mass - omega * vx;
        
M  = Fyf * obj.lf - Fyr * obj.lr;        
omega_dot = M / obj.Inertia;        

end

== matlab function P4_Model_Final/CarLateralDynamicsBodyFrame/TireForces ==
  data: alpha_f input; alpha_r input; Fyf output; obj parameter; Fyr output
function [Fyf, Fyr] = fcn(alpha_f, alpha_r, obj)

Fyf = min(obj.Fyfmax,obj.Calpha_f * alpha_f);
Fyr = min(obj.Fyrmax, obj.Calpha_r * alpha_r);
end

== matlab function P4_Model_Final/Braking/MATLAB Function ==
  data: Tbcap input; Tb output; v input; Tw input; w_wheel input
function Tb = fcn(Tbcap, v, Tw,w_wheel)
Tb = Tbcap * v/(abs(v)+0.001);
end

% wrong, more logic needs to be added to this
% try to find where to incorporate Tw and w_wheel into function

== matlab function P4_Model_Final/CarLateralDynamicsBodyFrame/TireSlip ==
  data: vy input size=1; vx input; delta_f input size=1; omega input; alpha_f output; obj parameter; alpha_r output
function [alpha_f, alpha_r] = fcn(vy,  vx, delta_f, omega, obj)


if abs(vx)> obj.vx_threshold1
      alpha_f = delta_f - (vy + omega * obj.lf) / vx;
      alpha_r = - (vy - omega * obj.lr) / vx;
else
      alpha_f = 0;
      alpha_r = 0;
end



end
